simulink model "package"  (R2018b)
settings: Solver=FixedStepDiscrete  StartTime=0.0  StopTime=10  FixedStep=Ts  RelTol=1e-3
PreLoadFcn:
  | Ts = 0.001;
InitFcn:
  | Ts = 0.001;
  | %mex controller.c;
undefined symbols (not defined in the file or in its folder): DiscIntNeverNeededParam, x2m
libraries: powerlib_meascontrol x6, motion x5, simulink x2, peGeneralControl x2
(part 1 of 2)
settings Model: Creator=Kamran  LastModifiedBy=Kamran

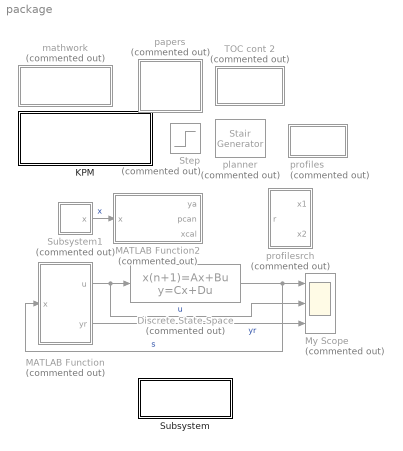
== system package ==
  Discrete State-Space : DiscreteStateSpace  Commented=on  A=A  B=B  C=C  D=D  SampleTime=-1  mask{Ts=Ts, n=3, int_type=off}
      mask prompts: Ts "Sample Time"; n "Order"; int_type "Simplified"
      mask init:
      | if int_type
      |     A = zeros(n);
      |     A(1:end-1, 2:end) = eye(n-1) * Ts;
      |     A = A + eye(n);
      | 
      |     B = zeros(n, 1);
      |     B(end) = Ts;
      | 
      |     C = eye(n);
      | 
      |     D = zeros(n, 1);
      | else
      |     syms ts
      |     B = sym(ones(n, 1));
      |     for i = 2:n+1
      |         B(i) = int(B(i-1), ts);
      |     end
      |     B = flip(B);
      |     A = sym(zeros(n));
      |     for i = 0:n-1
      |         tmp = sym(zeros(n));
      |         tmp(1:end-i, i+1:end) = eye(n-i) * B(n-i+1);
      |         A = A + tmp;
      |     end
      |     B = B(1:end-1);
      |     C = eye(n);
      |     D = zeros(n, 1);
      |     
      |     A = double(subs(A, ts, Ts));
      |     B = double(subs(B, ts, Ts));
      | end
  KPM : Subsystem
  MATLAB Function : MATLAB Function  Commented=on  TreatAsAtomicUnit=on  SystemSampleTime=Ts
  MATLAB Function2 : MATLAB Function  Commented=on  TreatAsAtomicUnit=on
  My Scope : Scope  Commented=on  NumInputPorts=3
  Step : Step  Commented=on  SampleTime=Ts
  Subsystem : Subsystem
  Subsystem1 : Subsystem  Commented=on
  TOC cont 2 : Subsystem  Commented=on
  mathwork : Subsystem  Commented=on
  papers : Subsystem  Commented=on
  planner : powerlib_meascontrol/Pulse & Signal Generators/Stair Generator  Commented=on  t=[0, 2, 5, 8]  e=[0, 1, 0.1, 0]  Ts=Ts
      settings: SourceProductName=Simscape Electrical
  profiles : Subsystem  Commented=on
  profilesrch : Subsystem  Commented=on  mask{x3p=3, x3m=-2, x2p=1, x2m=-2, Ts=Ts}
  wires:
  MATLAB Function/1(u) -> Discrete State-Space/1, My Scope/2  "u"
  Discrete State-Space/1 -> MATLAB Function/1(x), My Scope/1  "s"
  Subsystem1/1(x) -> MATLAB Function2/1(x)  "x"
  MATLAB Function/2(yr) -> My Scope/3  "yr"

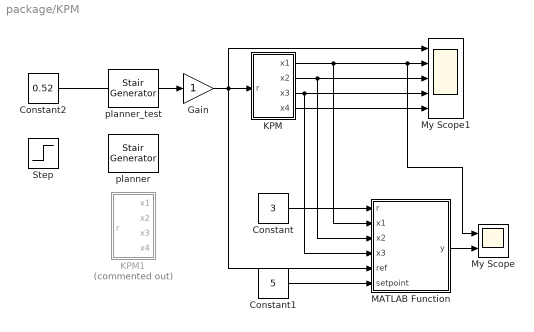
== system package/KPM ==
  Constant : Constant  Value=3
  Constant1 : Constant  Value=5
  Constant2 : Constant  Value=0.52
  Gain : Gain
  KPM : Subsystem  mask{x2mp=1, x2mn=1, x3mp=1.5, x3mn=1, x4m=3, ts=Ts}
      mask prompts: x2mp "x2m+"; x2mn "x2m-"; x3mp "x3m+"; x3mn "x3m-"
  KPM1 : Subsystem  Commented=on  mask{x2mp=0.5, x2mn=0.4, x3mp=0.5, x3mn=0.6, x4m=2, ts=Ts}
      mask prompts: x2mp "x2m+"; x2mn "x2m-"; x3mp "x3m+"; x3mn "x3m-"
  MATLAB Function : MATLAB Function  TreatAsAtomicUnit=on
  My Scope : Scope  NumInputPorts=2
  My Scope1 : Scope  NumInputPorts=5
  Step : Step  SampleTime=0
  planner : powerlib_meascontrol/Pulse & Signal Generators/Stair Generator  t=[0, 1, 1.3, 8]  e=[0, 1, 0.9, 0]  Ts=Ts
      settings: SourceProductName=Simscape Electrical
  planner_test : powerlib_meascontrol/Pulse & Signal Generators/Stair Generator  t=[0, 1, 2]  e=[0, 1,0.4]  Ts=Ts
      settings: SourceProductName=Simscape Electrical
  wires:
  KPM/4(x4) -> My Scope1/5
  Constant2/1 -> Gain/1
  KPM/2(x2) -> MATLAB Function/3(x2), My Scope1/3
  KPM/3(x3) -> MATLAB Function/4(x3), My Scope1/4
  KPM/1(x1) -> MATLAB Function/2(x1), My Scope/1, My Scope1/2
  MATLAB Function/1(y) -> My Scope/2
  Constant/1 -> MATLAB Function/1(r)
  Gain/1 -> MATLAB Function/5(ref), KPM/1(r), My Scope1/1
  Constant1/1 -> MATLAB Function/6(setpoint)

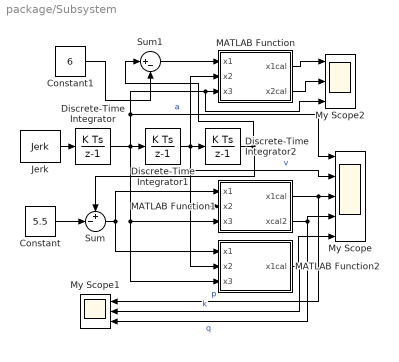
== system package/Subsystem ==
  Constant : Constant  Value=5.5
  Constant1 : Constant  Value=6
  Discrete-Time Integrator : DiscreteIntegrator  SampleTime=-1  ICPrevOutput=DiscIntNeverNeededParam  ICPrevScaledInput=DiscIntNeverNeededParam
  Discrete-Time Integrator1 : DiscreteIntegrator  SampleTime=-1  ICPrevOutput=DiscIntNeverNeededParam  ICPrevScaledInput=DiscIntNeverNeededParam
  Discrete-Time Integrator2 : DiscreteIntegrator  SampleTime=-1  ICPrevOutput=DiscIntNeverNeededParam  ICPrevScaledInput=DiscIntNeverNeededParam
  Jerk : motion/Profile Generators/Jerk  t0=1  x=6  v=1  a=0.5  j=3  Ts=Ts
  MATLAB Function : MATLAB Function  TreatAsAtomicUnit=on
  MATLAB Function1 : MATLAB Function  TreatAsAtomicUnit=on
  MATLAB Function2 : MATLAB Function  TreatAsAtomicUnit=on
  My Scope : Scope  NumInputPorts=5
  My Scope1 : Scope  NumInputPorts=3
  My Scope2 : Scope  NumInputPorts=3
  Sum : Sum  Inputs=+-|
  Sum1 : Sum  Inputs=|+-
  wires:
  Jerk/1 -> Discrete-Time Integrator/1
  Discrete-Time Integrator/1 -> My Scope2/3, MATLAB Function/3(x3), My Scope/1, MATLAB Function2/3(x3), MATLAB Function1/3(x3), Discrete-Time Integrator1/1  "a"
  Discrete-Time Integrator1/1 -> MATLAB Function/2(x2), MATLAB Function2/2(x2), MATLAB Function1/2(x2), My Scope/2, Discrete-Time Integrator2/1  "v"
  Discrete-Time Integrator2/1 -> Sum1/1, Sum/1
  MATLAB Function2/1(x1cal) -> My Scope/5, My Scope1/2  "k"
  MATLAB Function1/1(x1cal) -> My Scope1/1, My Scope/3  "p"
  Sum/1 -> MATLAB Function2/1(x1), MATLAB Function1/1(x1)
  Constant/1 -> Sum/2
  MATLAB Function1/2(xcal2) -> My Scope/4, My Scope1/3  "q"
  MATLAB Function/1(x1cal) -> My Scope2/1
  MATLAB Function/2(x2cal) -> My Scope2/2
  Sum1/1 -> MATLAB Function/1(x1)
  Constant1/1 -> Sum1/2

== system package/Subsystem1 ==
  Discrete State-Space : DiscreteStateSpace  A=A  B=B  C=C  D=D  SampleTime=-1  mask{Ts=Ts, n=3, int_type=on}
      mask prompts: int_type "Simplified"
      mask init: same as package/Discrete State-Space
  Jerk : motion/Profile Generators/Jerk  t0=0  x=8  v=2.5  a=10  j=3  Ts=Ts
  x : Outport
  wires:
  Jerk/1 -> Discrete State-Space/1
  Discrete State-Space/1 -> x/1

== system package/TOC cont 2 ==
  Constant : Constant
  Discrete-Time Integrator : DiscreteIntegrator  SampleTime=-1  LimitOutput=on  UpperSaturationLimit=2  LowerSaturationLimit=-2  ICPrevOutput=DiscIntNeverNeededParam  ICPrevScaledInput=DiscIntNeverNeededParam
  Discrete-Time Integrator1 : DiscreteIntegrator  SampleTime=-1  ICPrevOutput=DiscIntNeverNeededParam  ICPrevScaledInput=DiscIntNeverNeededParam
  My Scope1 : Scope  NumInputPorts=2
  TOC2 : MATLAB Function  TreatAsAtomicUnit=on
  wires:
  Discrete-Time Integrator1/1 -> TOC2/2(x1), My Scope1/1
  Discrete-Time Integrator/1 -> TOC2/3(x2), My Scope1/2, Discrete-Time Integrator1/1
  TOC2/1(u) -> Discrete-Time Integrator/1
  Constant/1 -> TOC2/1(v)

== system package/mathwork ==
  Acceleration : motion/Profile Generators/Acceleration  t0=1  x=3  v=1  a=2  Ts=Ts
  Derivative of Jerk : motion/Profile Generators/Derivative of Jerk  t0=1  x=4  v=1  a=2  j=3  d=4  Ts=Ts
  Discrete State-Space : DiscreteStateSpace  A=A  B=B  C=C  D=D  SampleTime=-1  mask{Ts=Ts, n=4, int_type=on}
      mask prompts: int_type "Simplified"
      mask init: same as package/Discrete State-Space
  Jerk : motion/Profile Generators/Jerk  t0=1  x=3  v=1  a=2  j=3  Ts=Ts
  My Scope3 : Scope
  wires:
  Discrete State-Space/1 -> My Scope3/1
  Derivative of Jerk/1 -> Discrete State-Space/1

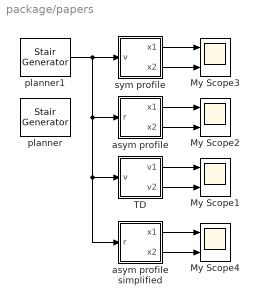
== system package/papers ==
  My Scope{1..4} (4 alike) : Scope  NumInputPorts=2
  TD : Subsystem  mask{x3m=3, x2mp=2, x2mn=2, w=1}
      mask prompts: x3m "x3 max"; x2mp "x2 max +"; x2mn "x2 max -"; w "w nominal"
  asym profile : Subsystem  mask{x3p=3, x3m=-3, x2p=2, x2m=-2, w=1, Ts=Ts}
      mask prompts: w "scale"
  asym profile simplified : Subsystem  mask{x3p=10, x3m=-3, x2p=1.5, x2m=-1, w=1, Ts=Ts}
      mask prompts: w "scale"
  planner : powerlib_meascontrol/Pulse & Signal Generators/Stair Generator  t=[0, 1, 5, 8]  e=[0, 1, 0.1, 0]  Ts=Ts
      settings: SourceProductName=Simscape Electrical
  planner1 : powerlib_meascontrol/Pulse & Signal Generators/Stair Generator  t=[0, 1, 5, 8]  e=[0, 1, 0, 0]  Ts=Ts
      settings: SourceProductName=Simscape Electrical
  sym profile : Subsystem  mask{x3m=3, x2m=2, w=1}
      mask prompts: x3m "x3 max"; x2m "x2 max"; w "w nominal"
  wires:
  asym profile/1(x1) -> My Scope2/1
  asym profile/2(x2) -> My Scope2/2
  planner1/1 -> asym profile/1(r), TD/1(v), asym profile simplified/1(r), sym profile/1(v)
  TD/1(v1) -> My Scope1/1
  TD/2(v2) -> My Scope1/2
  sym profile/1(x1) -> My Scope3/1
  sym profile/2(x2) -> My Scope3/2
  asym profile simplified/2(x2) -> My Scope4/2
  asym profile simplified/1(x1) -> My Scope4/1

== system package/profiles ==
  Subsystem2 : Subsystem  mask{P=6, V=1, A=2, J=3, Ts=Ts, d=1, w=2 * pi * 1500 / 60}
      mask prompts: w "w nominal"
      mask Display: disp('s-curve')
  Subsystem3 : Subsystem  mask{P=6, V=1, A=2, J=3, Ts=Ts, d=1}
      mask Display: disp('st-curve')
  acc_optimal : Subsystem
  hashem profile : Subsystem

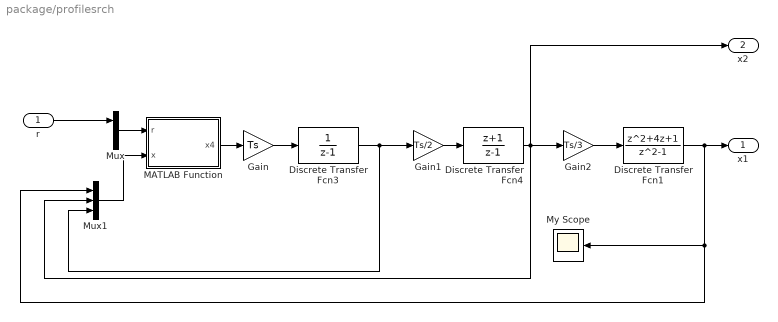
== system package/profilesrch ==
  r : Inport
  Discrete Transfer Fcn1 : DiscreteTransferFcn  Numerator=[1 4 1]  Denominator=[1 0 -1]
  Discrete Transfer Fcn3 : DiscreteTransferFcn  Denominator=[1 -1]
  Discrete Transfer Fcn4 : DiscreteTransferFcn  Numerator=[1 1]  Denominator=[1 -1]
  Gain : Gain  Gain=Ts
  Gain1 : Gain  Gain=Ts/2
  Gain2 : Gain  Gain=Ts/3
  MATLAB Function : MATLAB Function  TreatAsAtomicUnit=on
  Mux : Mux  Inputs=3
  Mux1 : Mux  Inputs=3
  My Scope : Scope
  x1 : Outport
  x2 : Outport  Port=2
  wires:
  r/1 -> Mux/1
  Gain/1 -> Discrete Transfer Fcn3/1
  Discrete Transfer Fcn3/1 -> Mux1/3, Gain1/1
  Gain1/1 -> Discrete Transfer Fcn4/1
  Discrete Transfer Fcn4/1 -> Mux1/2, x2/1, Gain2/1
  Gain2/1 -> Discrete Transfer Fcn1/1
  Discrete Transfer Fcn1/1 -> My Scope/1, Mux1/1, x1/1
  MATLAB Function/1(x4) -> Gain/1
  Mux/1 -> MATLAB Function/1(r)
  Mux1/1 -> MATLAB Function/2(x)

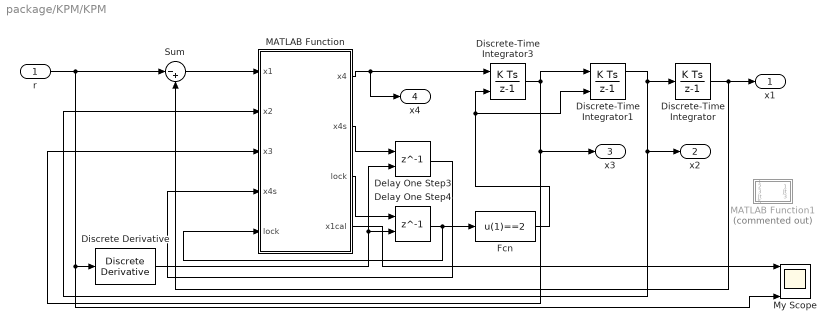
== system package/KPM/KPM ==
  r : Inport
  Delay One Step3 : Delay  DelayLength=1  InitialCondition=x4m  ExternalReset=Level
      settings: InputPortMap=u0,r5
  Delay One Step4 : Delay  DelayLength=1  ExternalReset=Level
      settings: InputPortMap=u0,r5
  Discrete Derivative : simulink/Discrete/Discrete Derivative  gainval=1.0  ICPrevScaledInput=0.0  OutMin=[]  OutMax=[]  OutDataType=fixdt(1, 16)  OutScaling=2^-10  DoSatur=off
  Discrete-Time Integrator : DiscreteIntegrator  SampleTime=-1  ICPrevOutput=DiscIntNeverNeededParam  ICPrevScaledInput=DiscIntNeverNeededParam
  Discrete-Time Integrator1 : DiscreteIntegrator  ExternalReset=level  InitialCondition=1  SampleTime=-1  LimitOutput=on  UpperSaturationLimit=x2mp  LowerSaturationLimit=-x2mn  ShowSaturationPort=on  ICPrevOutput=DiscIntNeverNeededParam  ICPrevScaledInput=DiscIntNeverNeededParam
  Discrete-Time Integrator3 : DiscreteIntegrator  ExternalReset=level  InitialCondition=-1  SampleTime=-1  LimitOutput=on  UpperSaturationLimit=x3mp  LowerSaturationLimit=-x3mn  ICPrevOutput=DiscIntNeverNeededParam  ICPrevScaledInput=DiscIntNeverNeededParam
  Fcn : Fcn  Expr=u(1)==2
  MATLAB Function : MATLAB Function  TreatAsAtomicUnit=on
  MATLAB Function1 : MATLAB Function  Commented=on  TreatAsAtomicUnit=on  mask{LoopTime=Ts, ACC=x3mp, DCC=x3mn, Vmax=x2m}
  My Scope : Scope  NumInputPorts=4
  Sum : Sum  Inputs=|-+
  x1 : Outport
  x2 : Outport  Port=2
  x3 : Outport  Port=3
  x4 : Outport  Port=4
  wires:
  Discrete-Time Integrator3/1 -> x3/1, MATLAB Function/3(x3), Discrete-Time Integrator1/1
  Delay One Step4/1 -> Fcn/1, MATLAB Function/5("lock ")
  MATLAB Function/2(x4s) -> Delay One Step3/1
  Discrete-Time Integrator1/1 -> Discrete-Time Integrator/1, x2/1, MATLAB Function/2(x2)
  r/1 -> My Scope/4, Discrete Derivative/1, Sum/1
  MATLAB Function/1(x4) -> Discrete-Time Integrator3/1, x4/1
  MATLAB Function/3(lock) -> Delay One Step4/1
  Discrete Derivative/1 -> Delay One Step4/2, Delay One Step3/2
  Discrete-Time Integrator/1 -> Sum/2, x1/1
  Sum/1 -> MATLAB Function/1(x1)
  Delay One Step3/1 -> MATLAB Function/4("x4s ")
  Fcn/1 -> Discrete-Time Integrator3/2, Discrete-Time Integrator1/2
  MATLAB Function/4(x1cal) -> My Scope/1

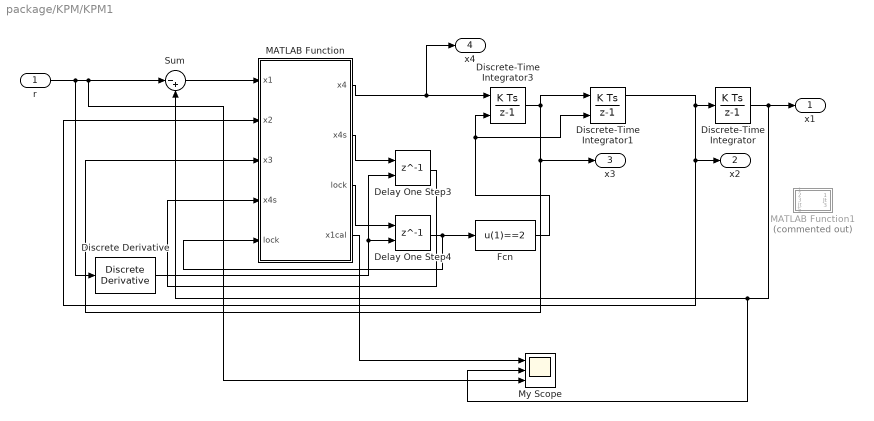
== system package/KPM/KPM1 ==
  r : Inport
  Delay One Step3 : Delay  DelayLength=1  InitialCondition=x4m  ExternalReset=Level
      settings: InputPortMap=u0,r5
  Delay One Step4 : Delay  DelayLength=1  ExternalReset=Level
      settings: InputPortMap=u0,r5
  Discrete Derivative : simulink/Discrete/Discrete Derivative  gainval=1.0  ICPrevScaledInput=0.0  OutMin=[]  OutMax=[]  OutDataType=fixdt(1, 16)  OutScaling=2^-10  DoSatur=off
  Discrete-Time Integrator : DiscreteIntegrator  SampleTime=-1  ICPrevOutput=DiscIntNeverNeededParam  ICPrevScaledInput=DiscIntNeverNeededParam
  Discrete-Time Integrator1 : DiscreteIntegrator  ExternalReset=level  SampleTime=-1  LimitOutput=on  UpperSaturationLimit=x2mp  LowerSaturationLimit=-x2mn  ShowSaturationPort=on  ICPrevOutput=DiscIntNeverNeededParam  ICPrevScaledInput=DiscIntNeverNeededParam
  Discrete-Time Integrator3 : DiscreteIntegrator  ExternalReset=level  SampleTime=-1  LimitOutput=on  UpperSaturationLimit=x3mp  LowerSaturationLimit=-x3mn  ICPrevOutput=DiscIntNeverNeededParam  ICPrevScaledInput=DiscIntNeverNeededParam
  Fcn : Fcn  Expr=u(1)==2
  MATLAB Function : MATLAB Function  TreatAsAtomicUnit=on
  MATLAB Function1 : MATLAB Function  Commented=on  TreatAsAtomicUnit=on  mask{LoopTime=Ts, ACC=x3mp, DCC=x3mn, Vmax=x2m}
  My Scope : Scope  NumInputPorts=3
  Sum : Sum  Inputs=|-+
  x1 : Outport
  x2 : Outport  Port=2
  x3 : Outport  Port=3
  x4 : Outport  Port=4
  wires:
  Discrete-Time Integrator3/1 -> x3/1, MATLAB Function/3(x3), Discrete-Time Integrator1/1
  Delay One Step4/1 -> Fcn/1, MATLAB Function/5("lock ")
  MATLAB Function/2(x4s) -> Delay One Step3/1
  Discrete-Time Integrator1/1 -> MATLAB Function/2(x2), x2/1, Discrete-Time Integrator/1
  r/1 -> My Scope/3, Sum/1, Discrete Derivative/1
  MATLAB Function/1(x4) -> x4/1, Discrete-Time Integrator3/1
  MATLAB Function/3(lock) -> Delay One Step4/1
  Discrete Derivative/1 -> Delay One Step4/2, Delay One Step3/2
  Discrete-Time Integrator/1 -> x1/1, My Scope/2, Sum/2
  Sum/1 -> MATLAB Function/1(x1)
  Delay One Step3/1 -> MATLAB Function/4("x4s ")
  Fcn/1 -> Discrete-Time Integrator3/2, Discrete-Time Integrator1/2
  MATLAB Function/4(x1cal) -> My Scope/1

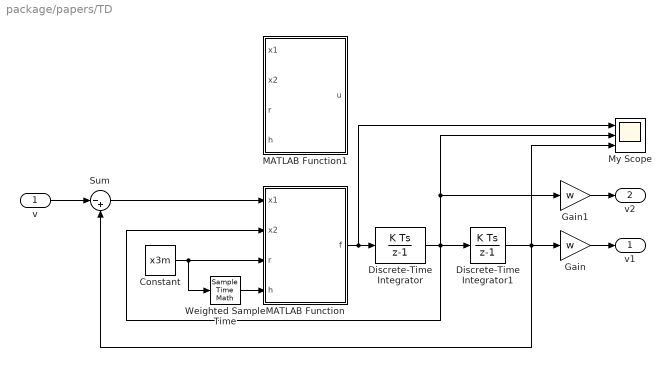
== system package/papers/TD ==
  v : Inport
  Constant : Constant  Value=x3m  SampleTime=-1
  Discrete-Time Integrator : DiscreteIntegrator  SampleTime=-1  LimitOutput=on  UpperSaturationLimit=x2mp  LowerSaturationLimit=-x2mn  ICPrevOutput=DiscIntNeverNeededParam  ICPrevScaledInput=DiscIntNeverNeededParam
  Discrete-Time Integrator1 : DiscreteIntegrator  SampleTime=-1  ICPrevOutput=DiscIntNeverNeededParam  ICPrevScaledInput=DiscIntNeverNeededParam
  Gain : Gain  Gain=w
  Gain1 : Gain  Gain=w
  MATLAB Function : MATLAB Function  TreatAsAtomicUnit=on
  MATLAB Function1 : MATLAB Function  TreatAsAtomicUnit=on
  My Scope : Scope  NumInputPorts=3
  Sum : Sum  Inputs=|-+
  Weighted Sample Time : SampleTimeMath  TsampMathOp=Ts Only
  v1 : Outport
  v2 : Outport  Port=2
  wires:
  Discrete-Time Integrator/1 -> MATLAB Function/2(x2), My Scope/2, Gain1/1, Discrete-Time Integrator1/1
  Discrete-Time Integrator1/1 -> My Scope/3, Sum/2, Gain/1
  Weighted Sample Time/1 -> MATLAB Function/4(h)
  Sum/1 -> MATLAB Function/1(x1)
  Constant/1 -> MATLAB Function/3(r), Weighted Sample Time/1
  MATLAB Function/1(f) -> My Scope/1, Discrete-Time Integrator/1
  Gain/1 -> v1/1
  Gain1/1 -> v2/1
  v/1 -> Sum/1

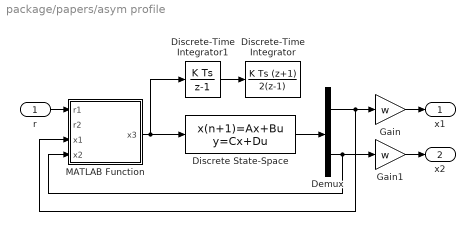
== system package/papers/asym profile ==
  r : Inport
  Demux : Demux  Outputs=2
  Discrete State-Space : DiscreteStateSpace  A=A  B=B  C=C  D=D  SampleTime=-1  mask{Ts=Ts, n=2, int_type=off}
      mask prompts: int_type "Simplified"
      mask init: same as package/Discrete State-Space
  Discrete-Time Integrator : DiscreteIntegrator  IntegratorMethod=Integration: Trapezoidal  SampleTime=-1  ICPrevOutput=DiscIntNeverNeededParam  ICPrevScaledInput=DiscIntNeverNeededParam
  Discrete-Time Integrator1 : DiscreteIntegrator  SampleTime=-1  ICPrevOutput=DiscIntNeverNeededParam  ICPrevScaledInput=DiscIntNeverNeededParam
  Gain : Gain  Gain=w
  Gain1 : Gain  Gain=w
  MATLAB Function : MATLAB Function  TreatAsAtomicUnit=on
  x1 : Outport
  x2 : Outport  Port=2
  wires:
  Discrete-Time Integrator1/1 -> Discrete-Time Integrator/1
  MATLAB Function/1(x3) -> Discrete State-Space/1, Discrete-Time Integrator1/1
  r/1 -> MATLAB Function/1(r1)
  Demux/1 -> Gain/1, MATLAB Function/3(x1)
  Demux/2 -> Gain1/1, MATLAB Function/4(x2)
  Gain/1 -> x1/1
  Gain1/1 -> x2/1
  Discrete State-Space/1 -> Demux/1

== system package/papers/asym profile simplified ==
  r : Inport
  Discrete-Time Integrator1 : DiscreteIntegrator  SampleTime=-1  LimitOutput=on  UpperSaturationLimit=x2p  LowerSaturationLimit=x2m  ICPrevOutput=DiscIntNeverNeededParam  ICPrevScaledInput=DiscIntNeverNeededParam
  Discrete-Time Integrator2 : DiscreteIntegrator  IntegratorMethod=Integration: Trapezoidal  SampleTime=-1  ICPrevOutput=DiscIntNeverNeededParam  ICPrevScaledInput=DiscIntNeverNeededParam
  Gain : Gain  Gain=w
  Gain1 : Gain  Gain=w
  MATLAB Function : MATLAB Function  TreatAsAtomicUnit=on
  Sum : Sum  Inputs=|-+
  x1 : Outport
  x2 : Outport  Port=2
  wires:
  Gain1/1 -> x2/1
  Gain/1 -> x1/1
  Discrete-Time Integrator1/1 -> MATLAB Function/2(x2), Gain1/1, Discrete-Time Integrator2/1
  Discrete-Time Integrator2/1 -> Sum/2, Gain/1
  r/1 -> Sum/1
  MATLAB Function/1(x3) -> Discrete-Time Integrator1/1
  Sum/1 -> MATLAB Function/1(x1)

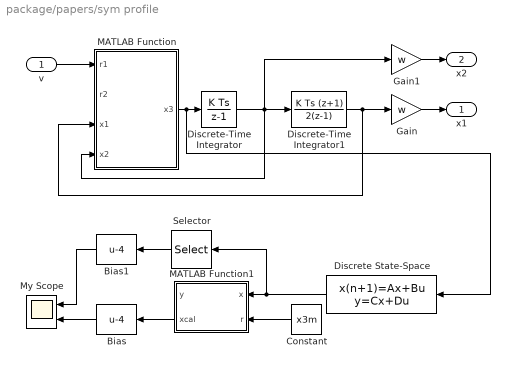
== system package/papers/sym profile ==
  v : Inport
  Bias : Bias  Bias=-4
  Bias1 : Bias  Bias=-4
  Constant : Constant  Value=x3m
  Discrete State-Space : DiscreteStateSpace  A=A  B=B  C=C  D=D  SampleTime=-1  mask{Ts=Ts, n=3, int_type=off}
      mask prompts: int_type "Simplified"
      mask init: same as package/Discrete State-Space
  Discrete-Time Integrator : DiscreteIntegrator  SampleTime=-1  ICPrevOutput=DiscIntNeverNeededParam  ICPrevScaledInput=DiscIntNeverNeededParam
  Discrete-Time Integrator1 : DiscreteIntegrator  IntegratorMethod=Integration: Trapezoidal  SampleTime=-1  ICPrevOutput=DiscIntNeverNeededParam  ICPrevScaledInput=DiscIntNeverNeededParam
  Gain : Gain  Gain=w
  Gain1 : Gain  Gain=w
  MATLAB Function : MATLAB Function  TreatAsAtomicUnit=on
  MATLAB Function1 : MATLAB Function  TreatAsAtomicUnit=on
  My Scope : Scope  NumInputPorts=2
  Selector : Selector  InputPortWidth=3  IndexOptions=Index vector (dialog)  Indices=1  OutputSizes=1
  x1 : Outport
  x2 : Outport  Port=2
  wires:
  Discrete-Time Integrator/1 -> Gain1/1, MATLAB Function/4(x2), Discrete-Time Integrator1/1
  Discrete-Time Integrator1/1 -> MATLAB Function/3(x1), Gain/1
  MATLAB Function/1(x3) -> Discrete State-Space/1, Discrete-Time Integrator/1
  Gain/1 -> x1/1
  Gain1/1 -> x2/1
  v/1 -> MATLAB Function/1(r1)
  Constant/1 -> MATLAB Function1/2(r)
  Discrete State-Space/1 -> Selector/1, MATLAB Function1/1(x)
  MATLAB Function1/2(xcal) -> Bias/1
  Selector/1 -> Bias1/1
  Bias1/1 -> My Scope/1
  Bias/1 -> My Scope/2

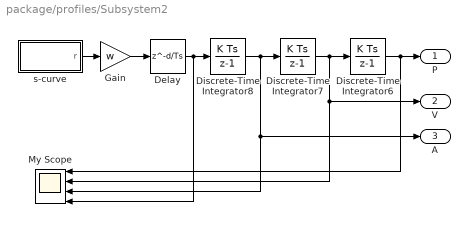
== system package/profiles/Subsystem2 ==
  Delay : Delay  DelayLength=d/Ts
  Discrete-Time Integrator6 : DiscreteIntegrator  SampleTime=-1  ICPrevOutput=DiscIntNeverNeededParam  ICPrevScaledInput=DiscIntNeverNeededParam
  Discrete-Time Integrator7 : DiscreteIntegrator  SampleTime=-1  ICPrevOutput=DiscIntNeverNeededParam  ICPrevScaledInput=DiscIntNeverNeededParam
  Discrete-Time Integrator8 : DiscreteIntegrator  SampleTime=-1  ICPrevOutput=DiscIntNeverNeededParam  ICPrevScaledInput=DiscIntNeverNeededParam
  Gain : Gain  Gain=w
  My Scope : Scope  NumInputPorts=4
  s-curve : MATLAB Function  TreatAsAtomicUnit=on  SystemSampleTime=Ts  mask{P=P, V=V, A=A, J=J, Ts=Ts}
  P : Outport
  V : Outport  Port=2
  A : Outport  Port=3
  wires:
  Delay/1 -> My Scope/4, Discrete-Time Integrator8/1
  Discrete-Time Integrator8/1 -> My Scope/3, A/1, Discrete-Time Integrator7/1
  Discrete-Time Integrator6/1 -> My Scope/1, P/1
  Discrete-Time Integrator7/1 -> My Scope/2, V/1, Discrete-Time Integrator6/1
  s-curve/1(r) -> Gain/1
  Gain/1 -> Delay/1

== system package/profiles/Subsystem3 ==
  Delay : Delay  DelayLength=d/Ts
  Discrete-Time Integrator6 : DiscreteIntegrator  SampleTime=-1  ICPrevOutput=DiscIntNeverNeededParam  ICPrevScaledInput=DiscIntNeverNeededParam
  Discrete-Time Integrator7 : DiscreteIntegrator  SampleTime=-1  ICPrevOutput=DiscIntNeverNeededParam  ICPrevScaledInput=DiscIntNeverNeededParam
  Discrete-Time Integrator8 : DiscreteIntegrator  SampleTime=-1  ICPrevOutput=DiscIntNeverNeededParam  ICPrevScaledInput=DiscIntNeverNeededParam
  My Scope : Scope  NumInputPorts=4
  st-curve : MATLAB Function  TreatAsAtomicUnit=on  mask{P=P, V=V, A=A, J=J, Ts=Ts}
  P : Outport
  A : Outport  Port=2
  wires:
  st-curve/1(r) -> Delay/1
  Discrete-Time Integrator7/1 -> Discrete-Time Integrator6/1, My Scope/3
  Discrete-Time Integrator6/1 -> P/1, My Scope/4
  Discrete-Time Integrator8/1 -> Discrete-Time Integrator7/1, A/1, My Scope/2
  Delay/1 -> Discrete-Time Integrator8/1, My Scope/1

== system package/profiles/acc_optimal ==
  Constant : Constant
  Constant1 : Constant  Value=2
  Constant2 : Constant  Value=Ts
  Delay One Step : Delay  DelayLength=1
  Delay One Step1 : Delay  DelayLength=1
  MATLAB Function : MATLAB Function  TreatAsAtomicUnit=on
  My Scope : Scope  NumInputPorts=3
  planner1 : powerlib_meascontrol/Pulse & Signal Generators/Stair Generator  t=[0, 1, 5, 8]  e=[0, 1, 0.1, 0]  Ts=Ts
      settings: SourceProductName=Simscape Electrical
  wires:
  MATLAB Function/1(acc_) -> My Scope/1
  Constant1/1 -> MATLAB Function/5(Am)
  Constant/1 -> MATLAB Function/4(Vm)
  Delay One Step1/1 -> My Scope/2, MATLAB Function/3(vel)
  MATLAB Function/3(pos_) -> Delay One Step/1
  MATLAB Function/2(vel_) -> Delay One Step1/1
  planner1/1 -> MATLAB Function/1(pd)
  Delay One Step/1 -> My Scope/3, MATLAB Function/2(pos)
  Constant2/1 -> MATLAB Function/6(dt)

== system package/profiles/hashem profile ==
  r : Inport
  Discrete-Time Integrator : DiscreteIntegrator  SampleTime=-1  ICPrevOutput=DiscIntNeverNeededParam  ICPrevScaledInput=DiscIntNeverNeededParam
  Discrete-Time Integrator1 : DiscreteIntegrator  SampleTime=-1  ICPrevOutput=DiscIntNeverNeededParam  ICPrevScaledInput=DiscIntNeverNeededParam
  Discrete-Time Integrator2 : DiscreteIntegrator  SampleTime=-1  ICPrevOutput=DiscIntNeverNeededParam  ICPrevScaledInput=DiscIntNeverNeededParam
  MATLAB Function2 : MATLAB Function  TreatAsAtomicUnit=on
  MATLAB Function3 : MATLAB Function  TreatAsAtomicUnit=on
  Sum : Sum  Inputs=|+-
  TD : Subsystem  mask{x3m=3, x2m=2, w=2 * pi * 120 / 60}
      mask prompts: x3m "x3 max"; x2m "x2 max"; w "w nominal"
  W : Outport
  A : Outport  Port=2
  wires:
  MATLAB Function2/3(x3dot) -> Discrete-Time Integrator2/1
  Discrete-Time Integrator2/1 -> MATLAB Function2/3(x3), MATLAB Function3/3(e3)
  MATLAB Function2/1(x1dot) -> Discrete-Time Integrator/1
  Discrete-Time Integrator/1 -> W/1, MATLAB Function2/1(x1), Sum/1
  MATLAB Function3/1(u) -> MATLAB Function2/4(u)
  Sum/1 -> MATLAB Function3/1(e1)
  MATLAB Function2/2(x2dot) -> Discrete-Time Integrator1/1
  TD/1(v1) -> Sum/2
  r/1 -> TD/1(v)
  Discrete-Time Integrator1/1 -> A/1, MATLAB Function3/2(e2), MATLAB Function2/2(x2)

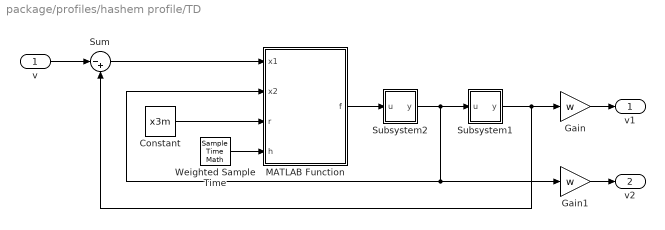
== system package/profiles/hashem profile/TD ==
  v : Inport
  Constant : Constant  Value=x3m  SampleTime=-1
  Gain : Gain  Gain=w
  Gain1 : Gain  Gain=w
  MATLAB Function : MATLAB Function  TreatAsAtomicUnit=on
  Subsystem1 : Subsystem  mask{sat=inf, x0=0}
      mask Display: droots([], [0], 1);
  Subsystem2 : Subsystem  mask{sat=x2m, x0=0}
      mask Display: droots([], [0], 1);
  Sum : Sum  Inputs=|-+
  Weighted Sample Time : SampleTimeMath  TsampMathOp=Ts Only
  v1 : Outport
  v2 : Outport  Port=2
  wires:
  Subsystem2/1(y) -> Subsystem1/1(u), Gain1/1, MATLAB Function/2(x2)
  Subsystem1/1(y) -> Sum/2, Gain/1
  v/1 -> Sum/1
  Weighted Sample Time/1 -> MATLAB Function/4(h)
  Sum/1 -> MATLAB Function/1(x1)
  Constant/1 -> MATLAB Function/3(r)
  MATLAB Function/1(f) -> Subsystem2/1(u)
  Gain/1 -> v1/1
  Gain1/1 -> v2/1

== system package/profiles/hashem profile/TD/Subsystem1 ==
  u : Inport
  Constant : Constant  Value=0
  Constant1 : Constant  Value=x0
  Integrator (Discrete or Continuous) : peGeneralControl/Integrator (Discrete or Continuous)  LabelModeActiveChoice=Discrete  ExternalReset=level  LimitType=Anti-windup  B=sat  A=-sat  Ts=-1
  y : Outport
  wires:
  Constant1/1 -> Integrator (Discrete or Continuous)/3
  u/1 -> Integrator (Discrete or Continuous)/1
  Constant/1 -> Integrator (Discrete or Continuous)/2
  Integrator (Discrete or Continuous)/1 -> y/1

== system package/profiles/hashem profile/TD/Subsystem2 ==
  u : Inport
  Constant : Constant  Value=0
  Constant1 : Constant  Value=x0
  Integrator (Discrete or Continuous) : peGeneralControl/Integrator (Discrete or Continuous)  LabelModeActiveChoice=Discrete  ExternalReset=level  LimitType=Anti-windup  B=sat  A=-sat  Ts=-1
  y : Outport
  wires:
  Integrator (Discrete or Continuous)/1 -> y/1
  Constant/1 -> Integrator (Discrete or Continuous)/2
  u/1 -> Integrator (Discrete or Continuous)/1
  Constant1/1 -> Integrator (Discrete or Continuous)/3

== matlab function package/papers/asym profile/MATLAB Function ==
  data: r1 input; r2 input; x1 input; x2 input; x3 output; Ts parameter; x2p parameter; x2m parameter; x3p parameter; x3m parameter
function x3 = guarino(r1, r2, x1, x2, Ts, x2p, x2m, x3p, x3m)

    y1 = x1 - r1;
    y2 = x2 - r2;

    z1 = y1/Ts^2 + y2/2/Ts;
    z2 = y2/Ts;

    z2p = (x2p - r2) / Ts;
    z2m = (x2m - r2) / Ts;

    z1p = -(floor(-z2p/x3m) + 1) * (z2p + floor(-z2p/x3m) * x3m/2);
    z1m = -(floor(-z2m/x3p) + 1) * (z2m + floor(-z2m/x3p) * x3p/2);

    gamma = sat(z1, z1p, z1m);

    if z1 <= 0
        alpha = x3m;
    else
        alpha = x3p;
    end

    m = floor(0.5 + sqrt(0.25 + 2*abs(gamma/alpha)));

    delta = z2 + gamma/m + (m-1)*alpha/2;

    if delta >= 0
        x3 = -x3m * sat(delta / x3m, -1, 1);
    else
        x3 = -x3p * sat(delta / x3p, -1, 1);
    end

end

function y = sat(u, low, high)
    y = max(low, min(high, u));
end

== matlab function package/profilesrch/MATLAB Function ==
  data: r input; x4 output; x input
function x4 = fcn(r, x)

T = 0.001;

x2p = +1; x2m = -1;
x3p = +2; x3m = -2;
x4p = +3; x4m = -3;

y = x - r;
W = [ T^3 -T^3 T^3/6
    0 T^2 -T^2/2
    0 0 T ];
z = W \ y;

r1 = r(1); r2 = r(2); r3 = r(3);
z1 = z(1); z2 = z(2); z3 = z(3);

z2p = (x2p - r2) / T^2 - r3 / 2*T;
z2m = (x2m - r2) / T^2 - r3 / 2*T;

z3p = x3p / T;
z3m = x3m / T;

z2bp = -ceil(-z3p/x4m) * (z3p + x4m/2*(ceil(-z3p/x4m) - 1));
z2bm = -ceil(-z3m/x4p) * (z3m + x4p/2*(ceil(-z3m/x4p) - 1));

d1 = z2 - z2p;
d2 = z2 - z2m;

gamma1 = sat(d1, z2bp, z2bm);
gamma2 = sat(d2, z2bp, z2bm);

if d1 <= 0
    kappa1 = x4m;
else
    kappa1 = x4p;
end

if d2 <= 0
    kappa2 = x4m;
else
    kappa2 = x4p;
end

m1 = floor(0.5 + sqrt(0.25 + 2*abs(gamma1/kappa1)));
m2 = floor(0.5 + sqrt(0.25 + 2*abs(gamma2/kappa2)));

sigma1 = -gamma1/m1 - (m1-1)*kappa1/2 - r3/T;
sigma2 = -gamma2/m2 - (m2-1)*kappa2/2 - r3/T;

[h, k, eta] = srch(z1, z2);

if eta > 0
    alpha = x4m;
    beta = x4p;
else
    alpha = x4p;
    beta = x4m;
end

sigma3 = 2 * z1 + (2*h+k-1) * z2 + k*(1-k^2)/6 * alpha ...
            + (2*h^3-3*h^2+h+3*h^2*k-3*h*k)/6 * beta;
sigma3 = -sigma3/h/(h+k);

sigma = sat(sigma3, sigma2, sigma1);
delta = z3 - sigma;

if delta >= 0
    x4 = -x4m * sat(delta/x4m, -1, 1);
else
    x4 = -x4p * sat(delta/x4p, -1, 1);
end

end

function [h, k, eta] = srch(z1, z2)
    r = 2; h = 0; k = 0; eta = 0;
    found = false;
    while ~found
        for h = 1:r-1
            k = r - h;
            eta = +1;
            if member(h, k, eta, [z1 z2])
                found = true;
            end
            eta = -1;
            if member(h, k, eta, [z1 z2])
                found = true;
            end
        end
        r = r + 1;
    end
end

function res = member(h, k, eta, z)
    p = eta * (Bhk(h+1, k-1) + Bhk(h, k)) / 2;
    v = eta * (Bhk(h, k+1) - Bhk(h, k));
    w = eta * (Bhk(h+1, k-1) - Bhk(h, k));
    A  =[w(1) 2*v(1)
        w(2) 2*v(2)];
    B = [2*z(1) -2*p(1)
         2*z(2) -2*p(2)];
    x = A\B;
    if abs(x(1)) <= 1 && 0 <= x(2) && x(2) <= 1
        res = true;
    else
        res = false;
    end
end

function B = Bhk(h, k)
    B = zeros(2, 1);
    B(1) = k*(k-1)*(k-2)/6 + k*(k-1)*h/2 + k*h*(h-1)/2 - h*(h-1)*(h-2)/6;
    B(2) = h*(h-1)/2-h*k-k*(k-1)/2;
end

function y = sat(u, low, high)
    y = max(low, min(high, u));
end

== matlab function package/papers/TD/MATLAB Function ==
  data: x1 input; f output; x2 input; r input; h input
function f = fhan(x1, x2, r, h)

    d = r * h^2;
    a0 = h * x2;
    y = x1 + a0;
    a1 = sqrt(d * (d + 8 * abs(y)));
    a2 = a0 + sign(y) * (a1 - d) / 2;
    sy = (sign(y + d) - sign(y - d)) / 2;
    a = (a0 + y - a2) * sy + a2;
    sa = (sign(a + d) - sign(a - d)) / 2;
    f = -r * (a / d - sign(a)) * sa - r * sign(a);

end

== matlab function package/MATLAB Function2 ==
  data: x input; ya output; pcan output; xcal output
function [ya, pcan, xcal] = straj(x)
    x1 = x(1) - 8; x2 = x(2); x3 = x(3);
    r = 3; h = 0.001; vm = 2.5;
    
    y1 = x1 + x3^3/3/r^2 + x3*abs(x2)/r;
    y2 = x1 + x3^3/3/r^2 - x3*abs(x2)/r;
    
    y3 = sign(x2) * (abs(x2) + x3^2/2/r);
    y4 = sign(x2) * (abs(x2) - x3^2/2/r);
    
    y5 = x2 + x3*abs(x3)/2/r;
    y6 = x2 - x3*abs(x3)/2/r;
    
    pcan = y3 * sqrt(abs(y3)/r);
    xcal = y1 + pcan;
    
%     y1 = -e + x3^3/3/r^2 + x2*x3/r;
%     y2 = -e + x3^3/3/r^2 - x2*x3/r;
%     y3 = x2 + x3^2/2/r;
%     y4 = x2 - x3^2/2/r;

    ya = [sqrt(abs(x2/r)) sqrt(abs(y3/r))];

%     P/V < (A/J + V/A)
%     V*J < A^2
%     ya = [abs(x2*r) x3^2];
%     ya = [abs(x1 / x2) abs(x3/r) + abs(x2/x3)];

%     ap = sqrt(vm/r);
%     ya(1) = (x3/r)*(x2+x3^2/6/r)+vm*(ap/2/r+vm/2/ap);
    
    x2max = x2+x3^2/2/r;
    x3max = sqrt(abs(x2max)*r);
    temp = ((-12*x2^3)*r^3 + (-36*x3^2*x2^2)*r^2 + (- 27*x3^4*x2 - 24*x3*x2*(x3max)^(3))*r - 16*x3^3*(x3max)^(3) - 6*x3^6)/(24*x3max^3*r^3);
    x4 = -1000*(x3-2/3*(x2+x3*0.001)^2/(x1+4/3*x2*0.001));
    ya(1) = temp;
    ya(2) = x4;
end

== matlab function package/KPM/MATLAB Function ==
  data: r input; y output; x1 input; x2 input; x3 input; ref input; setpoint input
function y = feasibility(r, x1, x2, x3, ref, setpoint)

    y1 = x1 + x3^3/3/r^2 + x3*abs(x2)/r;
    y3 = sign(x2) * (abs(x2) + x3^2/2/r);
    pcan = y3 * sqrt(abs(y3)/r);
    xcal = y1 + pcan;
    res = (sign(xcal - ref) * sign(xcal - setpoint)) >= 0;
    y = res && abs(setpoint) > abs(x1);
    
end

== matlab function package/papers/sym profile/MATLAB Function ==
  data: r1 input; x3 output; r2 input; x1 input; x2 input; x3m parameter; x2m parameter; Ts parameter
function x3 = morselli(r1, r2, x1, x2, x3m, x2m, Ts)

    y1 = x1 - r1;
    y2 = x2 - r2;
    z2 = y2 / Ts / x3m;
    z1 = (y1 / Ts + y2 / 2) / Ts / x3m;
    m = floor(0.5 + sqrt(1 + 8 * abs(z1)) / 2);
    sigma = z2 + z1 / m + 0.5 * (m - 1) * sign(z1);
    x3 = 0.5 + sign(x2 * sign(sigma) + x2m - Ts * x3m) / 2;
    x3 = -x3m * sat(sigma) * x3;

end

function u = sat(s)
    u = max(-1, min(+1, s));
end

== matlab function package/KPM/KPM1/MATLAB Function ==
  data: x1 input; x2 input; x3 input; x4s input; lock input; x4 output; x4s output; lock output; x3mp parameter; x3mn parameter; x2mp parameter; x2mn parameter; ts parameter; x1cal output
function [x4, x4s, lock, x1cal] = CalcFout(x1,x2,x3,x4s, lock, x3mp, x3mn, x2mp, x2mn, ts)
x1cal=0;
x2max = 0; x3max = 0;
if lock == 2
    x4 = 0;
    return
end

if x2 > 0
    x2m = x2mp;
else
    x2m = x2mn;
end

sx1 = sign(x1);
x3 = x3 * -sx1;
x2 = x2 * -sx1;
x1 = x1 * -sx1;

if sx1 > 0
    [x3mp, x3mn] = deal(x3mn, x3mp);
end

if x3 <= -x3mn
    x1cal = (1/24)*x3mn^3/x4s^2+x2^2/(2*x3mn) + x1;
else
    x2max = x2+x3^2/(x4s*2);
    x3max = min(x3mn,sqrt(abs(x2max)*x4s));
    if x3max == 0
        x1cal = 0;
    else
        x1cal = x3/x4s*(x2+(x3^2)/(3*x4s))+x2max*(x3max/x4s+x2max/x3max)/2 + x1;
    end
end

if x1cal > 0.0 || lock == 1
    if x3 <= -x3mn
        temp = -(1/12)*x3mn^3/(x4s^3);
    elseif  x3mn*x3mn < x2max * x4s
        temp = (-6*x2*(x3mn+x3)^2*x4s - x3^2*(6*x3mn^2+8*x3mn*x3+3*x3^2))/(12*x3mn*x4s^3);
    else
        temp = ((-12*x2^3)*x4s^3 + (-36*x3^2*x2^2)*x4s^2 + (- 27*x3^4*x2 - 24*x3*x2*(x3max)^(3))*x4s - 16*x3^3*(x3max)^(3) - 6*x3^6)/(24*x3max^3*x4s^3);
    end
    x4s = x4s - x1cal / temp;
    lock = 1;
    x4 = -1000*(x3-2/3*(x2+x3*0.001)^2/(x1+4/3*x2*0.001));
    if x4 < -x4s
        x4 = -x4s*1.0;
    end
    if x4 > x4s*1.1
        x4 = x4s*1.1;
    end
else
    x4 = x4s;
end

if x3 >= 0
    if x4 > 0
        if x2 + x3 * ts > x2m
            x4 = -x3 * ts;
        else
            dx2 = x3*x3/(2*x4s) + x3*ts/2;
            if x2 > x2m - dx2
                x4 = -(x3*x3)/( 2*(x2m-x2)- x3*0.001);
            else
                if x3 >= x3mp
                    x4 = 0;
                end
            end
        end
    end
    x4 = sat(x4, x4s * 1.1);
else
    if x3 > -x3mn || x4 > 0
        x4 = sat(x4, x4s * 1.5);
    else
        x4 = 0;
    end
end

if x2 < 0 && lock == 1
    lock = 2;
end

x4 = x4 * -sx1;

end

function o = sat(a,b)
    o = min(max(a, -b), b);
end

== matlab function package/KPM/KPM1/MATLAB Function1 ==
  data: Xout input; Vout input; Aout input; Jt input; Lock input; Jout output; Jt output; Lock output; ACC parameter; DCC parameter; Vmax parameter; LoopTime parameter
function [Jout, Jt, Lock]= CalcFout(Xout,Vout,Aout,Jt,Lock,ACC, DCC, Vmax, LoopTime)

vm = 0; am = 0;

if Lock == 2
    Jout = 0;
    return
end

sxout = sign(Xout);
Aout = Aout * -sxout;
Vout = Vout * -sxout;
Xout = Xout * -sxout;
if sxout > 0
    [ACC, DCC] = deal(DCC, ACC);
end

if Aout <= -DCC
    xcal = (1/24)*DCC^3/Jt^2+Vout^2/(2*DCC) + Xout;
else
    vm = Vout+Aout^2/(Jt*2);
    am = min(DCC,sqrt(abs(vm)*Jt));
    xcal = Aout/Jt*(Vout+(Aout^2)/(3*Jt))+vm*(am/Jt+vm/am)/2 + Xout;
end

if xcal > 0.0 || Lock == 1
    if Aout <= -DCC
        temp = -(1/12)*DCC^3/(Jt^3);
    elseif  DCC*DCC < vm * Jt
        temp = (-6*Vout*(DCC+Aout)^2*Jt - Aout^2*(6*DCC^2+8*DCC*Aout+3*Aout^2))/(12*DCC*Jt^3);
    else
        temp = ((-12*Vout^3)*Jt^3 + (-36*Aout^2*Vout^2)*Jt^2 + (- 27*Aout^4*Vout - 24*Aout*Vout*(am)^(3))*Jt - 16*Aout^3*(am)^(3) - 6*Aout^6)/(24*am^3*Jt^3);
    end
    Jt = Jt - xcal / temp;
    Lock = 1;
    Jout = -1000*(Aout-2/3*(Vout+Aout*0.001)^2/(Xout+4/3*Vout*0.001));
    if Jout < -Jt
        Jout = -Jt*1.0;
    end
    if Jout > Jt*1.1
        Jout = Jt*1.1;
    end
else
    Jout = Jt;
end

if Aout >= 0
    if Jout > 0
        if Vout + Aout * LoopTime > Vmax
            Jout = -Aout * LoopTime;
        else
            dv = Aout*Aout/(2*Jt) + Aout*LoopTime/2;
            if Vout > Vmax - dv
                Jout = -(Aout*Aout)/( 2*(Vmax-Vout)- Aout*0.001);
            else
                if Aout >= ACC
                    Jout = 0;
                    Aout = ACC;
                end
            end
        end
    end
    Jout = mysat(Jout, Jt * 1.1);
else
    if Aout > -DCC || Jout > 0
        Jout = mysat(Jout, Jt * 1.5);
    else
        Jout = 0;
        Aout = -DCC;
    end
end

if Vout < 0 && Lock == 1
    Lock = 2;
end

Jout = Jout * -sxout;

end

function o = mysat(a,b)
    o = min(max(a, -b), b);
end

== matlab function package/papers/TD/MATLAB Function1 ==
  data: x1 input; u output; x2 input; r input; h input
function u  = fst(x1, x2, r, h)

    d = r * h;
    d0 = h * d;
    y = x1 + h * x2;
    a0 = sqrt(d^2 + 8 * r * abs(y));
    if abs(y) > d0
        a = x2 + 0.5 * (a0 - d) * sign(y);
    else
        a = x2 + y / h;
    end
    if abs(a) > d
        u = -r * sign(a);
    else
        u = -r * a / d;
    end
    
end

== matlab function package/KPM/KPM/MATLAB Function1 ==
  data: Xout input; Vout input; Aout input; Jt input; Lock input; Jout output; Jt output; Lock output; ACC parameter; DCC parameter; Vmax parameter; LoopTime parameter
function [Jout, Jt, Lock]= CalcFout(Xout,Vout,Aout,Jt,Lock,ACC, DCC, Vmax, LoopTime)

vm = 0; am = 0;

if Lock == 2
    Jout = 0;
    return
end

sxout = sign(Xout);
Aout = Aout * -sxout;
Vout = Vout * -sxout;
Xout = Xout * -sxout;
if sxout > 0
    [ACC, DCC] = deal(DCC, ACC);
end

if Aout <= -DCC
    xcal = (1/24)*DCC^3/Jt^2+Vout^2/(2*DCC) + Xout;
else
    vm = Vout+Aout^2/(Jt*2);
    am = min(DCC,sqrt(abs(vm)*Jt));
    xcal = Aout/Jt*(Vout+(Aout^2)/(3*Jt))+vm*(am/Jt+vm/am)/2 + Xout;
end

if xcal > 0.0 || Lock == 1
    if Aout <= -DCC
        temp = -(1/12)*DCC^3/(Jt^3);
    elseif  DCC*DCC < vm * Jt
        temp = (-6*Vout*(DCC+Aout)^2*Jt - Aout^2*(6*DCC^2+8*DCC*Aout+3*Aout^2))/(12*DCC*Jt^3);
    else
        temp = ((-12*Vout^3)*Jt^3 + (-36*Aout^2*Vout^2)*Jt^2 + (- 27*Aout^4*Vout - 24*Aout*Vout*(am)^(3))*Jt - 16*Aout^3*(am)^(3) - 6*Aout^6)/(24*am^3*Jt^3);
    end
    Jt = Jt - xcal / temp;
    Lock = 1;
    Jout = -1000*(Aout-2/3*(Vout+Aout*0.001)^2/(Xout+4/3*Vout*0.001));
    if Jout < -Jt
        Jout = -Jt*1.0;
    end
    if Jout > Jt*1.1
        Jout = Jt*1.1;
    end
else
    Jout = Jt;
end

if Aout >= 0
    if Jout > 0
        if Vout + Aout * LoopTime > Vmax
            Jout = -Aout * LoopTime;
        else
            dv = Aout*Aout/(2*Jt) + Aout*LoopTime/2;
            if Vout > Vmax - dv
                Jout = -(Aout*Aout)/( 2*(Vmax-Vout)- Aout*0.001);
            else
                if Aout >= ACC
                    Jout = 0;
                    Aout = ACC;
                end
            end
        end
    end
    Jout = mysat(Jout, Jt * 1.1);
else
    if Aout > -DCC || Jout > 0
        Jout = mysat(Jout, Jt * 1.5);
    else
        Jout = 0;
        Aout = -DCC;
    end
end

if Vout < 0 && Lock == 1
    Lock = 2;
end

Jout = Jout * -sxout;

end

function o = mysat(a,b)
    o = min(max(a, -b), b);
end

== matlab function package/MATLAB Function ==
  data: u output; x input; yr output
function [u, yr] = TOC3(x)
x(1) = x(1) - 1; x1 = x(1); x2 = x(2); x3 = x(3);
r = 3; vm = 2.5; h = 0.001;

[y, xcal] = straj(x, r);
[xp] = simn(x, +r, h);
[yp, xcalp] = straj(xp, +r);

yr = [xcal 0 0 0 0];
yr(2) = x1+x2*sqrt(abs(x2/r));
yr(3) = (xcal/y(1));
yr(3) =  x2^3/x1^2;

% if abs(x1) < h && abs(x2) < h && abs(x3) < h
%     u  = 0;
%     return;
% end

% d = r * h;
% d0 = h * d;
% y = x1 + h * x2;
% if abs(xcal) > r*h*h
if xcal < 0
    if abs(yp(2)) >= vm
        u = morselli(x2 - vm * sign(x2), x3, r, h);
        yr(end-1) = 1;
    else
%         u = -r * sign(xcal);
        sigma = xcal * 5;
        u = -r * sat(sigma);
        yr(end-1) = 2;
    end
else
    u = morselli(x2, x3, r, h);
    yr(end-1) = 3;
    yr(end) = myround(abs(u), abs(log10(h^3))) == r;
end
end

function [xn] = simn(x, r, h)
    u = r * sign(x(2));
    x1 = x(1) + h * x(2) + h^2 * x(3) / 2 + h^3 * u / 6;
    x2 = x(2) + h * x(3) + h^2 * u / 2;
    x3 = x(3) + h * u;
    xn = [x1 x2 x3];
end

function [y, xcal] = straj(x, r)
    x1 = x(1); x2 = x(2); x3 = x(3);
    y1 = x1 + x3^3/3/r^2 + x3*abs(x2)/r;
    y2 = sign(x2) * (abs(x2) + x3^2/2/r);
    y3 = x2 + x3*abs(x3)/2/r;
    pcan = y2 * sqrt(abs(y2/r));
    xcal = y1 + pcan;
    y = [y1 y2 y3];
end

function x3 = morselli(x2, x3, r, h)
    z2 = x3 / h / r;
    z1 = (x2 / h + x3 / 2) / h / r;
    m = floor(0.5 + sqrt(0.25 + 2 * abs(z1)));
    sigma = z2 + z1 / m + 0.5 * (m - 1) * sign(z1);
    x3 = -r * sat(sigma);
end

function u = sat(s)
    u = max(-1, min(+1, s));
end

function y = myround(u, v)
    y = round(u * 10^v) / 10^v;
end

== matlab function package/TOC cont 2/TOC2 ==
  data: v input; u output; x1 input; x2 input
function u = TOC2(v, x1, x2)
    r = 3;
    h = eps;
    e = v - x1;
    y1 = -e + x2*abs(x2)/2/r;
    y2 = -e - x2*abs(x2)/2/r;
    
    if abs(y1) > h
        u = -r * sign(y1); %%%%%%%%%%%%%%%%%%%%%%%%%%%%%%%
    else
        if abs(y2) > h
            u = -r * sign(y2);
        else
            u = 0;
        end
    end
end

== matlab function package/papers/asym profile simplified/MATLAB Function ==
  data: x1 input; x2 input; x3 output; Ts parameter; x3p parameter; x3m parameter
function x3 = guarino(x1, x2, Ts, x3p, x3m)

    z1 = x1/Ts^2 + x2/2/Ts;
    z2 = x2/Ts;

    if z1 <= 0
        alpha = x3m;
    else
        alpha = x3p;
    end

    m = floor(0.5 + sqrt(0.25 + 2*abs(z1/alpha)));
    delta = z2 + z1/m + (m-1)*alpha/2;

    if delta >= 0
        gamma = x3m;
    else
        gamma = x3p;
    end
    
    x3 = -gamma * sat(delta / gamma);
    
end

function y = sat(u)
    y = max(-1, min(1, u));
end

== matlab function package/profiles/Subsystem2/s-curve ==
  data: r output; P parameter; V parameter; A parameter; J parameter; Ts parameter
function r = profile(P, V, A, J, Ts)

persistent t;
if isempty(t)
    t = 0;
else
    t = t + Ts;
end

if P/V < (A/J + V/A)
    b = A/J;
    V = A * (-b + sqrt(b^2 + 4*P/A)) / 2;
end

if V*J < A^2
    A = sqrt(J*V);
end

t1 = A/J;
t2 = V/A - A/J;
t3 = P/V - V/A - A/J;
t4 = t1;
t5 = t2;

t = round(t / Ts) * Ts;
t1 = round(t1 / Ts) * Ts;
t2 = round(t2 / Ts) * Ts;
t3 = round(t3 / Ts) * Ts;
t4 = round(t4 / Ts) * Ts;
t5 = round(t5 / Ts) * Ts;

K = 2*P/(t1*(t1+t2)*(t5+2*t4+2*t3+2*t1+t2));

if 0
elseif t < (t1)
    r = +K;
elseif t < (t1 + t2)
    r = 0;
elseif t < (2*t1 + t2)
    r = -K;
elseif t < (2*t1 + t2 + t3)
    r = 0;
elseif t < (2*t1 + t2 + t3 + t4)
    r = -K;
elseif t < (2*t1 + t2 + t3 + t4 + t5)
    r = 0;
elseif t < (2*t1 + t2 + t3 + 2*t4 + t5)
    r = K;
else
    r = 0;
end

end

== matlab function package/papers/sym profile/MATLAB Function1 ==
  data: x input; y output; r input; xcal output

function [y, xcal] = straj(x, r)
    x1 = x(1); x2 = x(2); x3 = x(3);
    y1 = x1 + x3^3/3/r^2 + x3*abs(x2)/r;
    y2 = sign(x2) * (abs(x2) + x3^2/2/r);
    y3 = x2 + x3*abs(x3)/2/r;
    pcan = y2 * sqrt(abs(y2/r));
    xcal = y1 + pcan;
    y = [y1 y2 y3];
end

== matlab function package/Subsystem/MATLAB Function1 ==
  data: x1 input; x1cal output; x2 input; x3 input; xcal2 output
function [x1cal,xcal2] = fcnp(x1,x2,x3)

x3mn = 1/2;
x4s = 3;
xcal2 =(1/24)*x3mn^3/x4s^2+x2^2/(2*x3mn) + x1;
if (x3 +x3mn) <= 0.001
    x1cal = (1/24)*x3mn^3/x4s^2+x2^2/(2*x3mn) + x1;
else
    x2max = x2+x3^2/(x4s*2);
    x3max = min(x3mn,sqrt(abs(x2max)*x4s));
    if x3max == 0
        x1cal = 0;
    else
        x1cal = x3/x4s*(x2+(x3^2)/(3*x4s))+x2max*(x3max/x4s+x2max/x3max)/2 + x1;
    end
end

== matlab function package/profiles/Subsystem3/st-curve ==
  data: r output; P parameter; V parameter; A parameter; J parameter; Ts parameter
function r = profile(P, V, A, J, Ts)

persistent t;
if isempty(t)
    t = 0;
else
    t = t + Ts;
end

if P/V < (3*A/2/J + V/A)
    a = 2*J;
    b = 3*A^2;
    c = -2*J*P*A;
    V = (-b + sqrt(b^2 - 4*a*c)) / (2*a);
end

if 2*J*V < 3*A^2
    A = sqrt(2*J*V/3);
end

t1 = 3*A/2/J;
t2 = V/A - t1;
t3 = P/V - V/A - t1;
t4 = t1;
t5 = t2;

t = round(t / Ts) * Ts;
t1 = round(t1 / Ts) * Ts;
t2 = round(t2 / Ts) * Ts;
t3 = round(t3 / Ts) * Ts;
t4 = round(t4 / Ts) * Ts;
t5 = round(t5 / Ts) * Ts;

K = 12*P/(t1^3*(t1+t2)*(t5+2*t4+2*t3+2*t1+t2));

if 0
elseif t < (t1)
    tt = t;
    ss = tt*(t1-tt);
    r = +K*ss;
elseif t < (t1 + t2)
    r = 0;
elseif t < (2*t1 + t2)
    tt = t - (t1 + t2);
    ss = tt*(t1-tt);
    r = -K*ss;
elseif t < (2*t1 + t2 + t3)
    r = 0;
elseif t < (2*t1 + t2 + t3 + t4)
    tt = t - (2*t1 + t2 + t3);
    ss = tt*(t1-tt);
    r = -K*ss;
elseif t < (2*t1 + t2 + t3 + t4 + t5)
    r = 0;
elseif t < (2*t1 + t2 + t3 + 2*t4 + t5)
    tt = t - (2*t1 + t2 + t3 + t4 + t5);
    ss = tt*(t1-tt);
    r = K*ss;
else
    r = 0;
end

end

== matlab function package/Subsystem/MATLAB Function2 ==
  data: x1 input; x1cal output; x2 input; x3 input
function x1cal = fcnk(x1,x2,x3)

x3mn = 1/2;
x4s = 3;

x2max = x2+x3^2/(x4s*2);
x3max = min(x3mn,sqrt(abs(x2max)*x4s));
if x3max == 0
    x1cal = x1;
else
    x1cal = x3/x4s*(x2+(x3^2)/(3*x4s))+x2max*(x3max/x4s+x2max/x3max)/2 + x1;
end

== matlab function package/profiles/acc_optimal/MATLAB Function ==
  data: acc_ output; vel_ output; pd input; pos_ output; pos input; vel input; Vm input; Am input; dt input
function [ acc_, vel_, pos_ ] = OTG( pd, pos, vel, Vm, Am, dt )
%Online trajectory generation with bounded vel and acc bounds
% @Yu Zhao
%   pd:     target position, default reach with 0 vel
%   pos:    current position
%   vel:    current velocity
%   Vm:     maximum velocity
%   Am:     maximum acceleration
%   dt:     sample time
dim = length(pd);
negDelta=pd(:)-pos(:);
ret = directionGeneral( negDelta );
% isotropy goalchanged axis limit
if length(Vm)==length(ret(:,1))
    VmI=min(abs(Vm(:))./abs(ret(:,1)));
elseif length(Vm)==1
    VmI=min(abs(Vm*ones(size(ret(:,1))))./abs(ret(:,1)));
end
if length(Am)==length(ret(:,1))
    AmI=min(abs(Am(:))./abs(ret(:,1)));
elseif length(Am)==1
    AmI=min(abs(Am*ones(size(ret(:,1))))./abs(ret(:,1)));
end
% otg code
delta_temp=pos(:)-pd(:);
tempv=zeros(dim,1);
tempa=zeros(dim,1);
for jj=1:dim
    x=[dot(delta_temp,ret(:,jj)),...
       dot(vel(:),ret(:,jj))];
    a=acc_control_optimal(x,VmI,...
                          AmI,dt);
    x_next=acc_dyn(x,a,dt);
    tempv(jj)=x_next(2);
    tempa(jj)=a;
end
vel_=ret*tempv;
acc_=ret*tempa;
pos_=pos(:)+vel(:)*dt+acc_(:)*dt^2/2;

function  [ ret ] = directionGeneral( Delta)
%get n orthonormal vectors from given displacement Delta
ret = RoughDirectionSet( Delta(:) );
n=size(ret,1);
ret(:,1)=ret(:,1)/norm(ret(:,1));
for ii=2:n
    vk=ret(:,ii);
    for jj=1:ii-1
        vk=vk-dot(ret(:,jj),vk)/norm(ret(:,jj))^2*ret(:,jj);
    end
    ret(:,ii)=vk/norm(vk);
end


function [ directionSet ] = RoughDirectionSet( Delta )
%from given delta generate rough directionset
%   directionSet: linear independent directions, start from resized Delta
v0 = Delta(:);
[~, ind] = max(abs(v0));
directionSet=zeros(length(v0));
directionSet(:,1)=v0;
% modify
if norm(v0,inf)==0
    directionSet(ind,1)=1;
end
for ii=ind+1:length(v0)
    directionSet(ii,ii+1-ind)=1;
end
m=length(v0)+1-ind;
for ii=1:ind-1
    directionSet(ii,ii+m)=1;
end

function [ a ] = acc_control_optimal( x, Vm, U, T)
yn=x(1);
ynd=x(2);
zn=1/(T*U)*(yn/T+ynd/2);
znd=ynd/(T*U);
m=floor((1+sqrt(1+8*abs(zn)))/2);
sigman=znd+zn/m+(m-1)/2*sign(zn);
a=-U*sat_fcn(sigman)*...
    (1+sign(...
    ynd*sign(sigman)+Vm-T*U...
    ))/2;

function [ y ]=sat_fcn(x)
y=min(max(x,-1),1);

function [ x_next ] = acc_dyn( x, a, dt )
ek=x(1);
vk=x(2);
ek_next=ek+vk*dt+1/2*a*dt^2;
vk_next=vk+a*dt;
x_next=[ek_next;vk_next];

== matlab function package/KPM/KPM/MATLAB Function ==
  data: x1 input; x2 input; x3 input; x4s input; lock input; x4 output; x4s output; lock output; x3mp parameter; x3mn parameter; x2mp parameter; x2mn parameter; ts parameter; x1cal output
function [x4, x4s, lock, x1cal] = CalcFout(x1,x2,x3,x4s, lock, x3mp, x3mn, x2mp, x2mn, ts)
x1cal=0;
x2max = 0; x3max = 0;
if lock == 2
    x4 = 0;
    return
end

if x2 > 0
    x2m = x2mp;
else
    x2m = x2mn;
end

sx1 = sign(x1);
x3 = x3 * -sx1;
x2 = x2 * -sx1;
x1 = x1 * -sx1;

if sx1 > 0
    [x3mp, x3mn] = deal(x3mn, x3mp);
end

% if x3 <= -x3mn
%     x1cal = (1/24)*x3mn^3/x4s^2+x2^2/(2*x3mn) + x1;
% else
    x2max = x2+x3^2/(x4s*2);
    x3max = min(x3mn,sqrt(abs(x2max)*x4s));
    if x3max == 0
        x1cal = 0;
    else
        x1cal = x3/x4s*(x2+(x3^2)/(3*x4s))+x2max*(x3max/x4s+x2max/x3max)/2 + x1;
    end
% end

if x1cal > 0.0 || lock == 1
    if x3 <= -x3mn
        temp = -(1/12)*x3mn^3/(x4s^3);
    elseif  x3mn*x3mn < x2max * x4s
        temp = (-6*x2*(x3mn+x3)^2*x4s - x3^2*(6*x3mn^2+8*x3mn*x3+3*x3^2))/(12*x3mn*x4s^3);
    else
        temp = ((-12*x2^3)*x4s^3 + (-36*x3^2*x2^2)*x4s^2 + (- 27*x3^4*x2 - 24*x3*x2*(x3max)^(3))*x4s - 16*x3^3*(x3max)^(3) - 6*x3^6)/(24*x3max^3*x4s^3);
    end
    x4s = x4s - x1cal / temp;
    lock = 1;
    x4 = -1000*(x3-2/3*(x2+x3*0.001)^2/(x1+4/3*x2*0.001));
    if x4 < -x4s
        x4 = -x4s*1.0;
    end
    if x4 > x4s*1.1
        x4 = x4s*1.1;
    end
else
    x4 = x4s;
end

if x3 >= 0
    if x4 > 0
        if x2 + x3 * ts > x2m
            x4 = -x3 * ts;
        else
            dx2 = x3*x3/(2*x4s) + x3*ts/2;
            if x2 > x2m - dx2
                x4 = -(x3*x3)/( 2*(x2m-x2)- x3*0.001);
            else
                if x3 >= x3mp
                    x4 = 0;
                end
            end
        end
    end
    x4 = sat(x4, x4s * 1.1);
else
    if x3 > -x3mn || x4 > 0
        x4 = sat(x4, x4s * 1.5);
    else
        x4 = 0;
    end
end

if x2 < 0 && lock == 1
    lock = 2;
end

x4 = x4 * -sx1;

end

function o = sat(a,b)
    o = min(max(a, -b), b);
end

== matlab function package/profiles/hashem profile/MATLAB Function2 ==
  data: x1 input; x2 input; x3 input; u input; x1dot output; x2dot output; x3dot output
function [x1dot,x2dot,x3dot] = fcn(x1,x2,x3,u)
x1dot=x2;
x2dot=x3;
x3dot=u;

== matlab function package/profiles/hashem profile/MATLAB Function3 ==
  data: e1 input; u output; e2 input; e3 input
function u = fcn(e1,e2,e3)
a=10;    
b=a;
c=a;

u= -a*b*c*e1 -((a+b)*c + a*b)*e2 -(a+b+c)*e3;

% eta=100;
% landa=150;
% sigma=1;
% s=e3+2*landa*e2+landa^2*e1;
% u=-2*landa*e3 - landa^2*e2 - eta*tanh(s/sigma) + xddd;
